simulink model "SF5_2_4_jc0531_2_A"  (R2016b)
settings: Solver=VariableStepAuto  StartTime=0.0  StopTime=10.0  RelTol=1e-3  EnableMultiTasking=on
settings Model: Creator=amyyang  LastModifiedBy=amyyang
settings DataIOCC: LimitDataPoints=on
settings OptimizationCC: LifeSpan=inf
settings DebuggingCC: AllowSymbolicDim=off  SFUnexpectedBacktrackingDiag=warning  SFNoUnconditionalDefaultTransitionDiag=warning  SFExecutionAtInitializationDiag=none
settings ModelReferenceCC: PropagateSignalLabelsOutOfModel=off
settings GRTTargetCC: TargetLangStandard=C89/C90 (ANSI)
settings ConfigComp: CovMetricSettings=dw  CovHtmlReporting=on  CovSaveCumulativeToWorkspaceVar=on  CovSaveSingleToWorkspaceVar=on  CovExternalEMLEnable=off

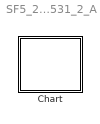
== system SF5_2_4_jc0531_2_A ==
  Chart : Stateflow chart  TreatAsAtomicUnit=on

== stateflow chart SF5_2_4_jc0531_2_A/Chart ==
  note: 跳转箭头不要与其它任何模型元素交叉，重叠。
  note: 互斥状态在任意一层必须有两个以上。
  note: 强烈建议默认箭头放在最左上角的明显位置
  state AA [parallel]
    settings: executionOrder=1
    state A
      state A1
      state A2
      (default) -> (junction 9)
      (junction 9) -> A1 [order 1]
      (junction 9) -> (junction 10) [order 2]
      A2 -> A1
      A1 -> A2
      (junction 10) -> A2
    (default) -> A
  state BB [parallel]
    settings: executionOrder=2
    state B
      state B1
      state B2
      B1 -> B2
      B2 -> B1
      (default) -> B2
    (default) -> B
  note: 这是为了说明默认跳转位置，因此未添加跳转条件
